simulink model "flightSimulation"  (R2021b)
settings: Solver=FixedStepAuto  StartTime=0  StopTime=end_time  FixedStep=0.005  RelTol=1e-3  EnableMultiTasking=on
undefined symbols (not defined in the file or in its folder): B, builder_switch, Earth, filter_switch, ft, initEuler, initPosLLA, inv_method, m, mass, s, sigbuilder_block, sw_turb, Ts, umax, umin, Vehicle, WGS84
libraries: slpidlib x8, dspsrcs4 x6, aerolibconvert2 x4, dspswit3 x3, aerolibanimutils x2, aerolibfltsims x2, shared6dof x1, aerolibtransform2 x1, qcatlib x1, aerolibwind2 x1, aerolibgravity2 x1, dspstat3 x1
(part 3 of 3)

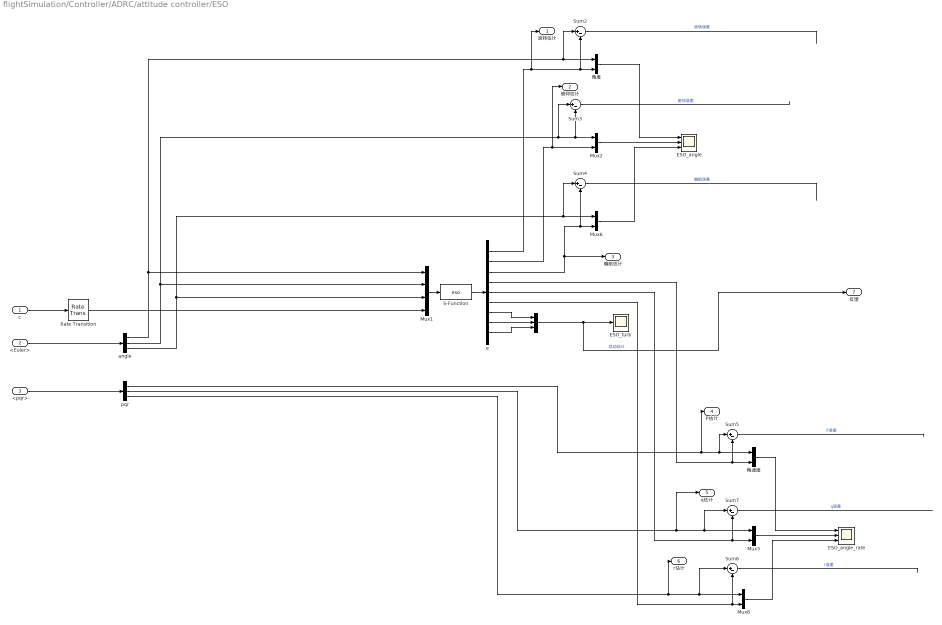
== system flightSimulation/Controller/ADRC/attitude controller/ESO ==
  c : Inport
  <Euler> : Inport  Port=2
  <pqr> : Inport  Port=3
  " " : Mux  Inputs=3
  ESO_angle : Scope  NumInputPorts=3
  ESO_angle_rate : Scope  NumInputPorts=3
  ESO_turb : Scope
  Mux1 : Mux
  Mux{2..3,6,8} (4 alike) : Mux  Inputs=2
  Rate Transition : RateTransition  OutPortSampleTime=0.01
  S-Function : S-Function  FunctionName=eso  SFunctionDeploymentMode=off  EnableBusSupport=off
  Sum{2..7} (6 alike) : Sum  Inputs=|+-
  angle : Demux  Outputs=3
  e : Demux  Outputs=9
  pqr : Demux  Outputs=3
  角度 : Mux  Inputs=2
  角速度 : Mux  Inputs=2
  滚转估计 : Outport  VectorParamsAs1DForOutWhenUnconnected=off
  俯仰估计 : Outport  Port=2  VectorParamsAs1DForOutWhenUnconnected=off
  偏航估计 : Outport  Port=3  VectorParamsAs1DForOutWhenUnconnected=off
  P估计 : Outport  Port=4  VectorParamsAs1DForOutWhenUnconnected=off
  q估计 : Outport  Port=5  VectorParamsAs1DForOutWhenUnconnected=off
  r估计 : Outport  Port=6  VectorParamsAs1DForOutWhenUnconnected=off
  反馈 : Outport  Port=7  VectorParamsAs1DForOutWhenUnconnected=off
  wires:
  e/1 -> 滚转估计/1, Sum2/2, 角度/2
  e/4 -> Sum5/2, 角速度/2
  pqr/1 -> P估计/1, Sum5/1, 角速度/1
  angle/1 -> Sum2/1, 角度/1, Mux1/1
  Sum4/1 -> ?  "偏航误差"
  e/8 -> " "/2
  angle/2 -> Mux2/1, Sum3/2, Sum3/1, Mux1/2
  e/6 -> Mux8/2, Sum6/2
  e/5 -> Sum7/2, Mux3/2
  angle/3 -> Mux6/1, Sum4/1, Mux1/3
  角速度/1 -> ESO_angle_rate/1
  Mux3/1 -> ESO_angle_rate/2
  e/3 -> 偏航估计/1, Sum4/2, Mux6/2
  Sum5/1 -> ?  "P误差"
  pqr/3 -> r估计/1, Sum6/1, Mux8/1
  角度/1 -> ESO_angle/1
  S-Function/1 -> e/1
  pqr/2 -> q估计/1, Sum7/1, Mux3/1
  <Euler>/1 -> angle/1
  Mux6/1 -> ESO_angle/3
  e/2 -> 俯仰估计/1, Mux2/2
  Mux2/1 -> ESO_angle/2
  e/7 -> " "/1
  Sum7/1 -> ?  "q误差"
  Mux1/1 -> S-Function/1
  Mux8/1 -> ESO_angle_rate/3
  e/9 -> " "/3
  Sum6/1 -> ?  "r误差"
  c/1 -> Rate Transition/1
  Sum3/1 -> ?  "俯仰误差"
  Sum2/1 -> ?  "滚转误差"
  <pqr>/1 -> pqr/1
  " "/1 -> 反馈/1, ESO_turb/1  "扰动估计"
  Rate Transition/1 -> Mux1/4

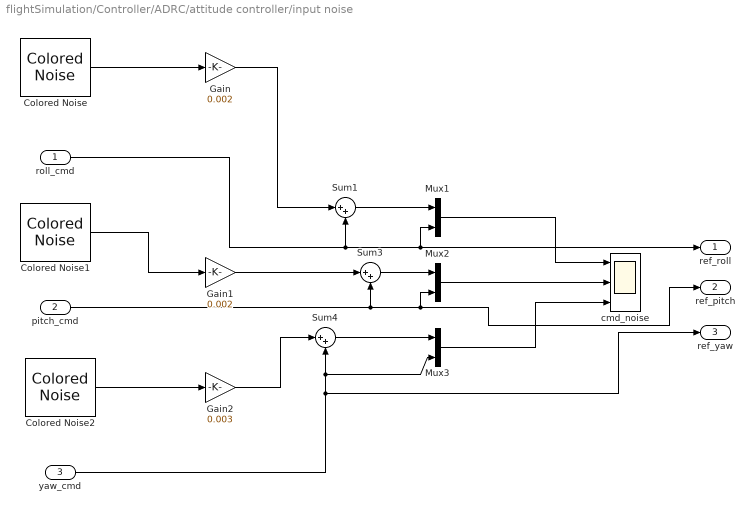
== system flightSimulation/Controller/ADRC/attitude controller/input noise ==
  roll_cmd : Inport
  pitch_cmd : Inport  Port=2
  yaw_cmd : Inport  Port=3
  Colored Noise : dspsrcs4/Colored Noise  Color=white  InverseFrequencyPower=1.55  BoundedOutput=off  NumChannels=1  OutputDataType=double  SamplesPerFrame=1  SampleTime=1  RandomStream=mt19937ar with seed  Seed=randperm(100000,1)  SimulateUsing=Interpreted execution
      settings: SourceProductBaseCode=DS
  Colored Noise1 : dspsrcs4/Colored Noise  Color=white  InverseFrequencyPower=1.55  BoundedOutput=off  NumChannels=1  OutputDataType=double  SamplesPerFrame=1  SampleTime=2  RandomStream=mt19937ar with seed  Seed=randperm(100000,1)  SimulateUsing=Interpreted execution
      settings: SourceProductBaseCode=DS
  Colored Noise2 : dspsrcs4/Colored Noise  Color=white  InverseFrequencyPower=1.55  BoundedOutput=off  NumChannels=1  OutputDataType=double  SamplesPerFrame=1  SampleTime=0.5  RandomStream=mt19937ar with seed  Seed=randperm(100000,1)  SimulateUsing=Interpreted execution
      settings: SourceProductBaseCode=DS
  Gain : Gain  Gain=0.002
  Gain1 : Gain  Gain=0.002
  Gain2 : Gain  Gain=0.003
  Mux1 : Mux  Inputs=2
  Mux2 : Mux  Inputs=2
  Mux3 : Mux  Inputs=2
  Sum1 : Sum  Inputs=|++
  Sum3 : Sum  Inputs=|++
  Sum4 : Sum  Inputs=|++
  cmd_noise : Scope  NumInputPorts=3
  ref_roll : Outport  VectorParamsAs1DForOutWhenUnconnected=off
  ref_pitch : Outport  Port=2  VectorParamsAs1DForOutWhenUnconnected=off
  ref_yaw : Outport  Port=3  VectorParamsAs1DForOutWhenUnconnected=off
  wires:
  roll_cmd/1 -> ref_roll/1, Mux1/2, Sum1/2
  pitch_cmd/1 -> ref_pitch/1, Mux2/2, Sum3/2
  yaw_cmd/1 -> ref_yaw/1, Sum4/2, Mux3/2
  Sum1/1 -> Mux1/1
  Sum4/1 -> Mux3/1
  Mux3/1 -> cmd_noise/3
  Mux2/1 -> cmd_noise/2
  Mux1/1 -> cmd_noise/1
  Colored Noise/1 -> Gain/1
  Colored Noise1/1 -> Gain1/1
  Colored Noise2/1 -> Gain2/1
  Sum3/1 -> Mux2/1
  Gain/1 -> Sum1/1
  Gain1/1 -> Sum3/1
  Gain2/1 -> Sum4/1

== system flightSimulation/Controller/ADRC/high controler/Subsystem ==
  q : Inport
  p : Inport  Port=2
  In3 : Inport  Port=3
  Divide : Product  Inputs=*/
  Gain : Gain  Gain=-1225^2/9.788
  Product : Product
  Saturation : Saturate  UpperLimit=-0.01  LowerLimit=-9.788*3
  Saturation1 : Saturate  UpperLimit=1  LowerLimit=0.5
  Sqrt : Sqrt  SaturateOnIntegerOverflow=on
  Trigonometric Function : Trigonometry  Operator=cos
  Trigonometric Function1 : Trigonometry  Operator=cos
  speed : Outport  VectorParamsAs1DForOutWhenUnconnected=off
  wires:
  Saturation1/1 -> Divide/2
  Trigonometric Function/1 -> Product/1
  In3/1 -> Divide/1
  Trigonometric Function1/1 -> Product/2
  p/1 -> Trigonometric Function/1
  Product/1 -> Saturation1/1
  q/1 -> Trigonometric Function1/1
  Divide/1 -> Saturation/1
  Gain/1 -> Sqrt/1
  Sqrt/1 -> speed/1
  Saturation/1 -> Gain/1

== matlab function flightSimulation/Sensor & Estimator/Filter/Kalman Filter/MATLAB Function ==
  settings: updateMethod=DISCRETE
  data: u input; y output
function y = fcn(u)

%   x_k是修正后的最有估计量X(k)，x_n是x_k的一步预测X(k+1|k)，作为下一时刻的输入，x_p上一时刻的一步预测X(k|k-1).

%   acc_m,mag_m,wgm分别是加速度计，磁力计(单位化)，陀螺仪的观测值，P是P（k|k-1）,dt是周期,PP是P(k+1|k),观测量为四元数和偏航角
    %% Q阵
%-6，0/-5，-1
    dt=0.01;
    acc_m=u(1:3)';
    wgm=u(4:6)';
    mag_m=u(7:9)'./norm(u(7:9));
    rad2deg=180/pi;
    Q_1 = 1e-5;
    Q_2 = 1e-5;
    Q_3 = 1e-5;
    Q_4 = 1e-5;
    Q_b1= 1e-5;
    Q_b2= 1e-5;
    Q_b3= 1e-5;
    Q = diag([Q_1 Q_2 Q_3 Q_4 Q_b1 Q_b2 Q_b3]);%系统噪声方差
    R=  [0.01    0           0       0;
        0       0.01      0       0; 
        0       0           0.01	0; 
        0	    0           0       0.001 ];

    persistent x P
    if isempty(x)
        euler_init = AccMag2Euler(-acc_m,mag_m).*rad2deg;
        q_init = euler2quaternion(euler_init);
        x = [q_init' 0 0 0];
    end
    if isempty(P)
        P =Q;
    end
    x_p=zeros(1,7);
    % 求一部预测
    F = zeros(7,7);
    wx = wgm(1);
    wy = wgm(2);
    wz = wgm(3);
    q0 = x(1);
    q1 = x(2);
    q2 = x(3);
    q3 = x(4);
    b_x = x(5);
    b_y = x(6);
    b_z = x(7);
    W_X = [0           -(wx-b_x)   -(wy-b_y)   -(wz-b_z);
           (wx-b_x)        0        wz-b_z     -(wy-b_y);
           (wy-b_y)    -(wz-b_z)       0        (wx-b_x);
           (wz-b_z)     (wy-b_y)   -(wx-b_x)       0];
    F(1:4,1:4) = 0.5 * W_X;
    F(1:4,5:7) = [q1  q2  q3;
                  -q0 q3  -q2;
                  -q3 -q0 q1;
                  q2  -q1 -q0];
    G = eye(7,7);
    tao = G*dt;
    Phi = (eye(7,7) + F * dt);   
    Temp = tao*Q*tao';
    H = zeros(4,7);
    H(1:4,1:4) = [2*q2 -2*q3 2*q0 -2*q1;
                  -2*q1 -2*q0 -2*q3  -2*q2;
                  -2*q0  2*q1 2*q2 -2*q3;
                  2*q3*(1-2*(q3^2+q2^2))/((1-2*(q3^2+q2^2))^2+4*(q2*q1+q0*q3)^2) 2*q2*(1-2*(q3^2+q2^2))/((1-2*(q3^2+q2^2))^2+4*(q2*q1+q0*q3)^2) (2*q1*(1-2*(q3^2+q2^2))+4*q2*(q1*q2+q0*q3))/((1-2*(q3^2+q2^2))^2+4*(q2*q1+q0*q3)^2) (2*q0*(1-2*(q3^2+q2^2))+4*q3*(q0*q3+q1*q2))/((1-2*(q3^2+q2^2))^2+4*(q2*q1+q0*q3)^2)];
    PP = Phi*P*Phi' + Temp;
    PP = (PP+PP')/2;
    x_p(1:4) = x(1:4) + (0.5 * dt * W_X * x(1:4)')';
    x_p(5:7) = x(5:7);
    q_p = x_p(1:4);
    q0 = q_p(1);
    q1 = q_p(2);
    q2 = q_p(3);
    q3 = q_p(4);
    %% 观测值的欧拉角
    euler_angle = AccMag2Euler(-acc_m,mag_m);
    yaw = euler_angle(3);
    Obs_value = [(acc_m./norm(acc_m))';yaw];%% 观测测量值00-
    
    Obs_value_p = zeros(4,1);%%预测的观测值
    Obs_value_p(1) = -2 * (q1 * q3 - q0 * q2);
    Obs_value_p(2) = -2 * (q2 * q3 + q0 * q1);
    Obs_value_p(3) = -(q0^2 - q1^2 - q2^2 + q3^2);
    Obs_value_p(4) = atan2(2*(q1*q2 + q0*q3),q0^2+q1^2-q2^2-q3^2);
    
    %% 观测矩阵
    error = Obs_value - Obs_value_p;
    if(error(4)>pi) 
        error(4) = error(4) - 2*pi;
    end
    if(error(4)<-pi) 
        error(4) = error(4) + 2*pi;
    end
    K = PP*H'/(H*PP*H'+R);
    x = x_p + (K * (error))';
    x(1:4) = x(1:4)./norm(x(1:4));
    P = (eye(7,7)-K*H)*PP;
    y=x';

== matlab function flightSimulation/Controller/ADRC/attitude controller/MATLAB Function ==
  data: x1_d input; u_r output; x2_d input; x1 input; x2 input
function u_r = NLSEF_yaw(x1_d,x2_d,x1,x2)
e1=x1_d-x1;
if e1<-pi
    a1=e1+2*pi;
elseif e1>=pi
    a1=e1-2*pi;
else   
    a1=e1;
end
e2=x2_d-x2;
% kp=0.5;kd=0.5;% 限11
% kp=1;kd=1; % 限20
kp=0.25;kd=0.25;% 噪声
alfa1=0.75;alfa2=1.5;
delta=0.1;
u_r = kp*fal(a1,alfa1,delta)+kd*fal(e2,alfa2,delta); 
% kp=0.5;kd=0.5;
% u_r = kp*a1+kd*e2;   % 控制输出
end

== matlab function flightSimulation/Controller/ADRC/attitude controller/MATLAB Function2 ==
  data: x1_d input; u_q output; x2_d input; x1 input; x2 input
function u_q = NLSEF_pitch(x1_d,x2_d,x1,x2)
e1=x1_d-x1;
e2=x2_d-x2;
% kp=1;kd=1.5;% 限11
% kp=1.5;kd=2;% 限20
kp=0.5;kd=0.5;% 噪声
alfa1=0.75;alfa2=1.5;
delta=0.1;
u_q = kp*fal(e1,alfa1,delta)+kd*fal(e2,alfa2,delta);   % 控制输出
% kp=0.4;kd=0.4;
% u_q = kp*e1+kd*e2;   % 控制输出
end

== matlab function flightSimulation/Controller/ADRC/attitude controller/MATLAB Function3 ==
  data: x1_d input; u_p output; x2_d input; x1 input; x2 input
function u_p = NLSEF_roll(x1_d,x2_d,x1,x2)
e1=x1_d-x1;
e2=x2_d-x2;
% kp=1;kd=1.5;% 限11
% kp=1.5;kd=2;% 限20
kp=0.5;kd=0.5;% 噪声
alfa1=0.75;alfa2=1.5;
delta=0.1;
u_p = kp*fal(e1,alfa1,delta)+kd*fal(e2,alfa2,delta);   % 控制输出
% kp=0.4;kd=0.4;
% u_p = kp*e1+kd*e2;   % 控制输出
end

== matlab function flightSimulation/Controller/PID/MATLAB Function ==
  data: u input; y output
function y = Eulerrate2pqr(u)
Roll=u(4);
Pitch=u(5);
Q=[1    sin(Roll)*tan(Pitch)    cos(Roll)*tan(Pitch);
   0        cos(Roll)               -sin(Roll);
   0    sin(Roll)*sec(Pitch)    cos(Roll)*sec(Pitch)];
y = Q\[u(1);u(2);u(3)];

== matlab function flightSimulation/Controller/PID/MATLAB Function1 ==
  data: u input; y output
function y = Yawcontrol(u)
if u<-pi
    a=u+2*pi;
elseif u>=pi
    a=u-2*pi;
else   
    a=u;
end
y = a;
